simulink model "pendule_inv_etu"  (R2022a)
settings: Solver=VariableStepAuto  StartTime=0.0  StopTime=100.0  RelTol=1e-3
values from neighbouring files (symbols this model uses):
  g = 9.81    [simu_pendule_inv_capteur_etu.m]    (also in simu_pendule_inv_etu.m)
  l = 10    [simu_pendule_inv_capteur_etu.m]    (also in simu_pendule_inv_etu.m)
  ue = 0    [simu_pendule_inv_capteur_etu.m]    (also in simu_pendule_inv_etu.m)
  x0 = [pi/20 0]'    [simu_pendule_inv_capteur_etu.m]    (also in simu_pendule_inv_etu.m)
  xe = [0 0]'    [simu_pendule_inv_capteur_etu.m]    (also in simu_pendule_inv_etu.m)
settings Model: Creator=acanon  LastModifiedBy=acanon

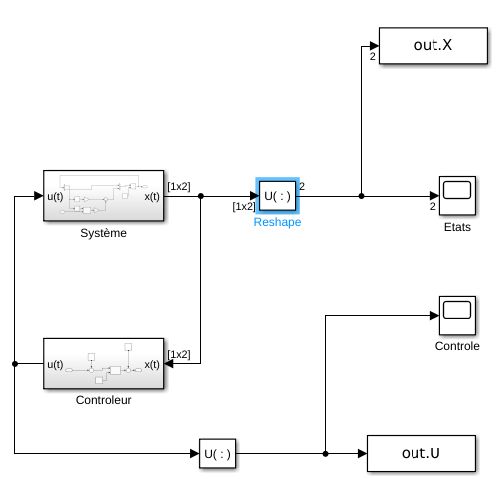
[thumbnail: Simulink's stored preview of the top-level diagram]
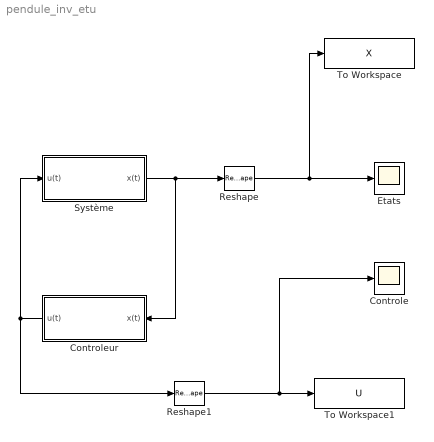
== system pendule_inv_etu ==
  Controle : Scope
  Controleur : Subsystem
  Etats : Scope
  Reshape : Reshape
  Reshape1 : Reshape
  Système : Subsystem
  To Workspace : ToWorkspace  VariableName=X  SaveFormat=Timeseries  SampleTime=-1
  To Workspace1 : ToWorkspace  VariableName=U  SaveFormat=Timeseries  SampleTime=-1
  wires:
  Controleur/1(u(t)) -> Système/1(u(t)), Reshape1/1
  Système/1(x(t)) -> Reshape/1, Controleur/1(x(t))
  Reshape/1 -> To Workspace/1, Etats/1
  Reshape1/1 -> Controle/1, To Workspace1/1

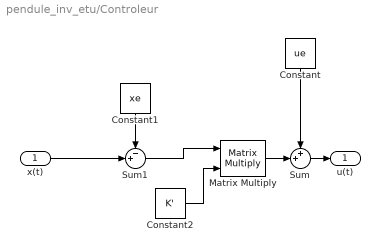
== system pendule_inv_etu/Controleur ==
  x(t) : Inport
  Constant : Constant  Value=ue
  Constant1 : Constant  Value=xe
  Constant2 : Constant  Value=K'  VectorParams1D=off
  Matrix Multiply : Product  Multiplication=Matrix(*)
  Sum : Sum  Inputs=++|
  Sum1 : Sum  Inputs=-+|
  u(t) : Outport
  wires:
  Constant/1 -> Sum/1
  x(t)/1 -> Sum1/2
  Sum/1 -> u(t)/1
  Matrix Multiply/1 -> Sum/2
  Constant1/1 -> Sum1/1
  Constant2/1 -> Matrix Multiply/2
  Sum1/1 -> Matrix Multiply/1

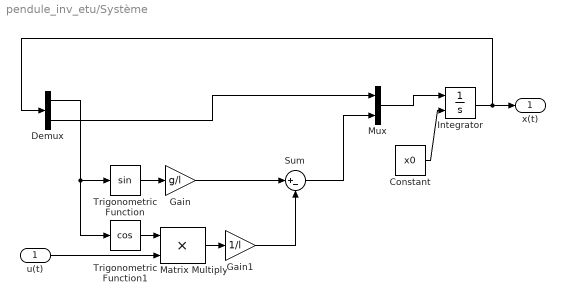
== system pendule_inv_etu/Système ==
  u(t) : Inport
  Constant : Constant  Value=x0
  Demux : Demux  Outputs=2
  Gain : Gain  Gain=g/l
  Gain1 : Gain  Gain=1/l
  Integrator : Integrator  InitialConditionSource=external
  Matrix Multiply : Product
  Mux : Mux  Inputs=2
  Sum : Sum  Inputs=|+-
  Trigonometric Function : Trigonometry
  Trigonometric Function1 : Trigonometry  Operator=cos
  x(t) : Outport
  wires:
  Trigonometric Function/1 -> Gain/1
  u(t)/1 -> Matrix Multiply/2
  Trigonometric Function1/1 -> Matrix Multiply/1
  Matrix Multiply/1 -> Gain1/1
  Gain/1 -> Sum/1
  Gain1/1 -> Sum/2
  Mux/1 -> Integrator/1
  Constant/1 -> Integrator/2
  Integrator/1 -> Demux/1, x(t)/1
  Demux/1 -> Trigonometric Function/1, Trigonometric Function1/1
  Demux/2 -> Mux/1
  Sum/1 -> Mux/2
